simulink model "MatlabModel"  (R2024a)
settings: Solver=ode14x  StartTime=0.0  StopTime=8  RelTol=1e-3
libraries: spsIGBTDiodeLib x4, spsSeriesRLCBranchLib x4, simulink x3, spsCurrentMeasurementLib x2, spsVoltageMeasurementLib x2, spsControlledVoltageSourceLib x1, sps_lib x1
settings Model: PacingRate=0.320000  Creator=user  LastModifiedBy=Arkebuzz

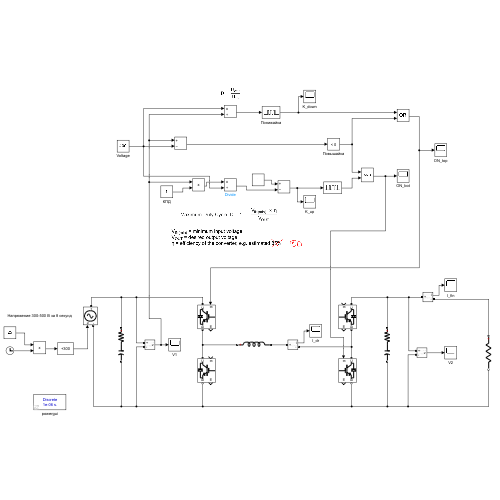
[thumbnail: Simulink's stored preview of the top-level diagram]
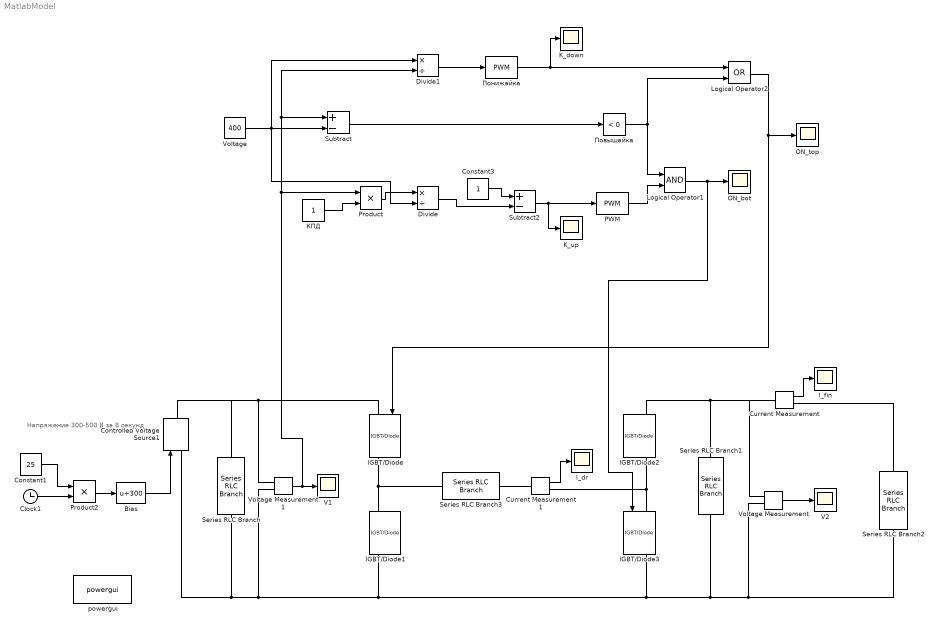
== system MatlabModel ==
  note: Напряжение 300-500 В за 8 секунд
  Bias : Bias  Bias=300  SaturateOnIntegerOverflow=off
  Clock1 : Clock
  Constant1 : Constant  Value=25
  Constant3 : Constant
  Controlled Voltage Source1 : spsControlledVoltageSourceLib/Controlled Voltage Source  Initialize=on  Source_Type=DC  Amplitude=0  Phase=0  Frequency=0  Measurements=None
  Current Measurement : spsCurrentMeasurementLib/Current Measurement  PhasorSimulation=off  OutputType=Complex  PSBequivalent=0
  Current Measurement1 : spsCurrentMeasurementLib/Current Measurement  PhasorSimulation=off  OutputType=Complex  PSBequivalent=0
  Divide : Product  Inputs=*/
  Divide1 : Product  Inputs=*/
  IGBT/Diode{,1..3} (4 alike) : spsIGBTDiodeLib/IGBT//Diode  Ron=1e-3  Rs=1e5  Cs=inf  Measurements=on
  I_dr : Scope
  I_fin : Scope
  K_down : Scope
  K_up : Scope
  Logical Operator1 : Logic  AllPortsSameDT=off  OutDataTypeStr=boolean
  Logical Operator2 : Logic  Operator=OR  AllPortsSameDT=off  OutDataTypeStr=boolean
  ON_bot : Scope
  ON_top : Scope
  PWM : simulink/Discontinuities/PWM  DisableCoverage=on  Period=3.34e-4  InitialDelay=0  DisallowZeroDutyCycle=off  RunAtFixedTimeIntervals=on  SampleTime=1e-6
  Product : Product
  Product2 : Product
  Series RLC Branch : spsSeriesRLCBranchLib/Series RLC Branch  LConnTagsString=__new0  RConnTagsString=__new0  BranchType=RC  Resistance=0.01  Inductance=1e-3  SetiL0=off  InitialCurrent=0  Capacitance=1e-2  Setx0=off  InitialVoltage=0  Measurements=None
  Series RLC Branch1 : spsSeriesRLCBranchLib/Series RLC Branch  LConnTagsString=__new0  RConnTagsString=__new0  BranchType=RC  Resistance=0.001  Inductance=1e-3  SetiL0=off  InitialCurrent=0  Capacitance=1e-2  Setx0=off  InitialVoltage=0  Measurements=None
  Series RLC Branch2 : spsSeriesRLCBranchLib/Series RLC Branch  LConnTagsString=__new0  RConnTagsString=__new0  BranchType=R  Resistance=5  Inductance=1e-3  SetiL0=off  InitialCurrent=0  Capacitance=1000e-6  Setx0=off  InitialVoltage=0  Measurements=None
  Series RLC Branch3 : spsSeriesRLCBranchLib/Series RLC Branch  LConnTagsString=__new0  RConnTagsString=__new0  BranchType=L  Resistance=1  Inductance=0.002  SetiL0=on  InitialCurrent=0  Capacitance=1e-6  Setx0=off  InitialVoltage=0  Measurements=None
  Subtract : Sum  Inputs=+-
  Subtract2 : Sum  Inputs=+-
  V1 : Scope
  V2 : Scope
  Voltage : Constant  Value=400
  Voltage Measurement : spsVoltageMeasurementLib/Voltage Measurement  PhasorSimulation=off  OutputType=Complex  PSBequivalent=0
  Voltage Measurement1 : spsVoltageMeasurementLib/Voltage Measurement  PhasorSimulation=off  OutputType=Complex  PSBequivalent=0
  powergui : sps_lib/powergui  Priority=1  SimulationMode=Discrete  SampleTime=1e-6  frequency=60  Iterations=50  frequencyindice=0  Pbase=100e6  ErrMax=1e-4  UnitsV=kV  UnitsW=MW  buscounter=0  FunctionMessages=off  echomessages=off  EnableUseOfTLC=off  CurrentSourceSwitches=off  DisableSnubberDevices=off  DisableRonSwitches=off  DisableVfSwitches=off  DisplayEquations=off  AutomaticDiscreteSolvers=off  SolverType=Tustin/Backward Euler (TBE)  Interpol=off  ExternalGateDelay=off  methode=off  Ts=100  x0status=blocks  SPID=on  SwTol=0  HookPort=off  NonlinearTolerance=1e-4  nMaxIteration=100  ContinueOnMaxIteration=off  RestoreLinks=warning  ResistiveCurrentMeasurement=off  Frange=[0:2:500]  Ylog=off  Xlog=on  ShowGrid=off  save=off  variable=ZData  structure=0  ZoomFFT=off  StartTime=0.0  cycles=1  DisplayStyle=1  fundamental=60  FreqAxis=off  MaxFrequency=1000  frequencyindicesteady=1  RmsSteady=1  display=off
  КПД : Constant
  Повышайка : simulink/Logic and Bit Operations/Compare To Constant  relop=<  const=0  OutDataTypeStr=boolean
  Понижайка : simulink/Discontinuities/PWM  DisableCoverage=on  Period=3.34e-4  InitialDelay=0  DisallowZeroDutyCycle=off  RunAtFixedTimeIntervals=on  SampleTime=1e-6
  wires:
  Current Measurement/1 -> I_fin/1
  Voltage Measurement1/1 -> V1/1, Product/1, Divide1/2, Subtract/1
  Voltage/1 -> Divide/2, Divide1/1, Subtract/2
  Subtract/1 -> Повышайка/1
  Повышайка/1 -> Logical Operator1/1, Logical Operator2/2
  Voltage Measurement/1 -> V2/1
  Logical Operator2/1 -> IGBT/Diode/1, ON_top/1
  Current Measurement1/1 -> I_dr/1
  КПД/1 -> Product/2
  Product/1 -> Divide/1
  Constant3/1 -> Subtract2/1
  Divide/1 -> Subtract2/2
  Subtract2/1 -> K_up/1, PWM/1
  PWM/1 -> Logical Operator1/2
  Clock1/1 -> Product2/2
  Bias/1 -> Controlled Voltage Source1/1
  Constant1/1 -> Product2/1
  Product2/1 -> Bias/1
  Logical Operator1/1 -> IGBT/Diode3/1, ON_bot/1
  Divide1/1 -> Понижайка/1
  Понижайка/1 -> K_down/1, Logical Operator2/1
  connections:
  IGBT/Diode/LConn1 -- Controlled Voltage Source1/RConn1 -- Series RLC Branch/LConn1 -- Voltage Measurement1/LConn1
  Series RLC Branch1/RConn1 -- Series RLC Branch2/RConn1 -- Voltage Measurement/LConn2 -- IGBT/Diode1/RConn1 -- Voltage Measurement1/LConn2 -- Controlled Voltage Source1/LConn1 -- Series RLC Branch/RConn1 -- IGBT/Diode3/RConn1
  IGBT/Diode/RConn1 -- Series RLC Branch3/LConn1 -- IGBT/Diode1/LConn1
  IGBT/Diode2/RConn1 -- IGBT/Diode3/LConn1 -- Current Measurement1/RConn1
  IGBT/Diode2/LConn1 -- Current Measurement/LConn1 -- Voltage Measurement/LConn1 -- Series RLC Branch1/LConn1
  Current Measurement/RConn1 -- Series RLC Branch2/LConn1
  Series RLC Branch3/RConn1 -- Current Measurement1/LConn1
